simulink model "DCAC_conv_VSM"  (R2025a)
settings: Solver=VariableStepAuto  StartTime=0.0  StopTime=10.0  RelTol=1e-3
undefined symbols (not defined in the file): Cf, Fi, Grid_op_VCVSC, Grid_op_VSM, Grid_opDC_VSM, Grid_opVCVSC, Ki_w, Kic, Kiv, Kp_id, Kp_theta, Kp_w, Kpc, Kpv, Lc, Lf, mp, nq, Preffast, Rc, Rf, t_step, Tf, VI_L, VI_R, WOF_Tf
libraries: simulink x3
(part 3 of 3)

== system DCAC_conv_VSM/VSM/VCC/dynamic_limiting/VI/WOF_d ==
  In1 : Inport
  Gain : Gain  Gain=iTf
  I : Integrator  InitialConditionSource=external  InitialCondition=Grid_op_VCVSC.op.States(16).x'
  Sum : Sum  Inputs=+-|
  Sum4 : Sum  Inputs=|+-
  Out1 : Outport
  wires:
  Gain/1 -> I/1
  Sum4/1 -> Gain/1
  In1/1 -> I/2, Sum/1, Sum4/1
  I/1 -> Sum/2, Sum4/2
  Sum/1 -> Out1/1

== system DCAC_conv_VSM/VSM/VCC/dynamic_limiting/VI/WOF_q ==
  In1 : Inport
  Gain : Gain  Gain=iTf
  I : Integrator  InitialConditionSource=external  InitialCondition=Grid_op_VCVSC.op.States(17).x'
  Sum : Sum  Inputs=+-|
  Sum4 : Sum  Inputs=|+-
  Out1 : Outport
  wires:
  Gain/1 -> I/1
  Sum4/1 -> Gain/1
  In1/1 -> I/2, Sum/1, Sum4/1
  I/1 -> Sum/2, Sum4/2
  Sum/1 -> Out1/1

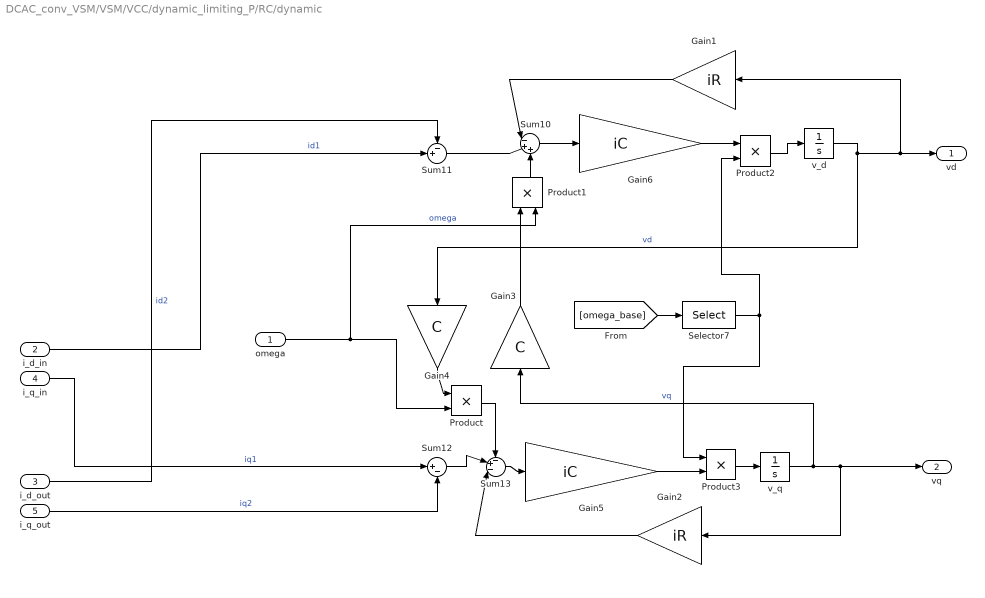
== system DCAC_conv_VSM/VSM/VCC/dynamic_limiting_P/RC/dynamic ==
  omega : Inport
  i_d_in : Inport  Port=2
  i_d_out : Inport  Port=3
  i_q_in : Inport  Port=4
  i_q_out : Inport  Port=5
  Gain1 : Gain  Gain=iR
  Gain2 : Gain  Gain=iR
  Gain3 : Gain  Gain=C
  Gain4 : Gain  Gain=C
  Gain5 : Gain  Gain=iC
  Gain6 : Gain  Gain=iC
  Product{,1..3} (4 alike) : Product
  Selector7 : Selector  InputPortWidth=length(fref.ref_units)  IndexOptions=Index vector (dialog)  Indices=block_fref  OutputSizes=1
  Sum10 : Sum  Inputs=|-++
  Sum11 : Sum  Inputs=-+|
  Sum12 : Sum  Inputs=|+-
  Sum13 : Sum  Inputs=-+-|
  v_d : Integrator  InitialCondition=Grid_opDC_VSM.vd_c
  v_q : Integrator  InitialCondition=Grid_opDC_VSM.vq_c
  vd : Outport
  vq : Outport  Port=2
  wires:
  Gain5/1 -> Product3/2
  Product3/1 -> v_q/1
  Selector7/1 -> Product3/1, Product2/2
  Product2/1 -> v_d/1
  Gain6/1 -> Product2/1
  [omega_base] -> Selector7/1
  i_q_out/1 -> Sum12/2  "iq2"
  i_q_in/1 -> Sum12/1  "iq1"
  i_d_out/1 -> Sum11/1  "id2"
  i_d_in/1 -> Sum11/2  "id1"
  v_d/1 -> Gain1/1, vd/1, Gain4/1  "vd"
  Sum12/1 -> Sum13/2
  Gain1/1 -> Sum10/1
  Sum13/1 -> Gain5/1
  omega/1 -> Product1/2, Product/2  "omega"
  Sum11/1 -> Sum10/2
  Product/1 -> Sum13/1
  Gain2/1 -> Sum13/3
  Gain4/1 -> Product/1
  Product1/1 -> Sum10/3
  v_q/1 -> Gain3/1, Gain2/1, vq/1  "vq"
  Gain3/1 -> Product1/1
  Sum10/1 -> Gain6/1

== system DCAC_conv_VSM/VSM/VCC/dynamic_limiting_P/RC/static ==
  omega : Inport
  i_d_in : Inport  Port=2
  i_d_out : Inport  Port=3
  i_q_in : Inport  Port=4
  i_q_out : Inport  Port=5
  Constant : Constant  Value=iR.^2
  Constant1 : Constant
  Divide : Product  Inputs=*/
  Gain : Gain  Gain=C
  Gain1 : Gain  Gain=iR
  Gain2 : Gain  Gain=iR
  Product{,1..5} (6 alike) : Product
  Sum : Sum  Inputs=|++
  Sum1 : Sum  Inputs=|-+
  Sum2 : Sum  Inputs=|+-
  Sum3 : Sum  Inputs=|++
  Sum4 : Sum  Inputs=|-+
  vd : Outport
  vq : Outport  Port=2
  wires:
  i_q_out/1 -> Sum2/2  "iq2"
  i_d_out/1 -> Sum2/1  "iq1"
  i_q_in/1 -> Sum1/1  "id2"
  i_d_in/1 -> Sum1/2  "id1"
  omega/1 -> Gain/1  "omega"
  Sum3/1 -> vd/1  "vd"
  Sum4/1 -> vq/1  "vq"
  Constant/1 -> Sum/1
  Sum/1 -> Divide/2
  Gain/1 -> Product2/2, Product/2, Product/1
  Product/1 -> Sum/2
  Constant1/1 -> Divide/1
  Sum1/1 -> Product1/1, Product4/1  "id"
  Sum2/1 -> Gain2/1, Product3/2  "iq"
  Gain1/1 -> Product1/2
  Divide/1 -> Product5/1, Gain1/1, Product2/1
  Product1/1 -> Sum3/1
  Product3/1 -> Sum3/2
  Product2/1 -> Product4/2, Product3/1
  Product4/1 -> Sum4/1
  Gain2/1 -> Product5/2
  Product5/1 -> Sum4/2

== system DCAC_conv_VSM/VSM/VCC/dynamic_limiting_P/RC/static omega ==
  i_d_in : Inport
  i_d_out : Inport  Port=2
  i_q_in : Inport  Port=3
  i_q_out : Inport  Port=4
  Gain : Gain  Gain=1./(iR.^2+C.^2)
  Gain2 : Gain  Gain=1./(iR.^2+C.^2)
  Gain3 : Gain  Gain=iR
  Gain4 : Gain  Gain=C
  Gain5 : Gain  Gain=iR
  Gain6 : Gain  Gain=C
  Sum : Sum  Inputs=|++
  Sum1 : Sum  Inputs=|+-
  Sum2 : Sum  Inputs=|+-
  Sum4 : Sum  Inputs=|-+
  vd : Outport
  vq : Outport  Port=2
  wires:
  Sum/1 -> vd/1
  Sum4/1 -> vq/1
  Gain5/1 -> Sum4/2
  Gain4/1 -> Sum4/1
  Gain6/1 -> Sum/2
  Gain3/1 -> Sum/1
  Gain2/1 -> Gain5/1, Gain6/1
  Gain/1 -> Gain3/1, Gain4/1
  i_d_out/1 -> Sum1/2
  i_d_in/1 -> Sum1/1  "id"
  i_q_out/1 -> Sum2/2  "iq2"
  Sum2/1 -> Gain2/1  "iq"
  Sum1/1 -> Gain/1  "id"
  i_q_in/1 -> Sum2/1  "iq1"

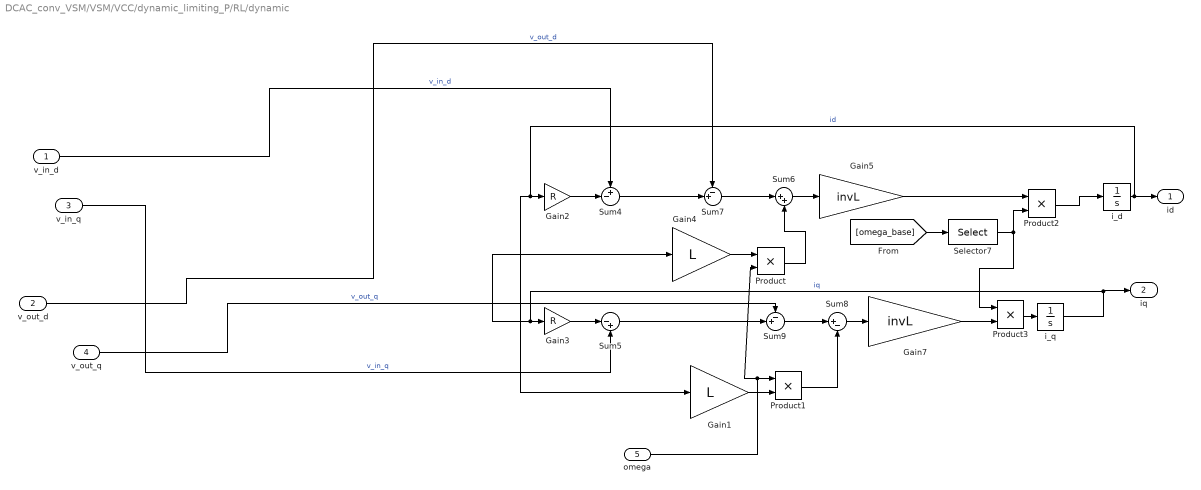
== system DCAC_conv_VSM/VSM/VCC/dynamic_limiting_P/RL/dynamic ==
  v_in_d : Inport
  v_out_d : Inport  Port=2
  v_in_q : Inport  Port=3
  v_out_q : Inport  Port=4
  omega : Inport  Port=5
  Gain1 : Gain  Gain=L
  Gain2 : Gain  Gain=R
  Gain3 : Gain  Gain=R
  Gain4 : Gain  Gain=L
  Gain5 : Gain  Gain=invL
  Gain7 : Gain  Gain=invL
  Product{,1..3} (4 alike) : Product
  Selector7 : Selector  InputPortWidth=length(fref.ref_units)  IndexOptions=Index vector (dialog)  Indices=block_fref  OutputSizes=1
  Sum4 : Sum  Inputs=+-|
  Sum5 : Sum  Inputs=|-+
  Sum6 : Sum  Inputs=|++
  Sum7 : Sum  Inputs=-+|
  Sum8 : Sum  Inputs=|+-
  Sum9 : Sum  Inputs=-+|
  i_d : Integrator  InitialCondition=Grid_opDC_VSM.id_l
  i_q : Integrator  InitialCondition=Grid_opDC_VSM.iq_l
  id : Outport
  iq : Outport  Port=2
  wires:
  Product3/1 -> i_q/1
  [omega_base] -> Selector7/1
  Selector7/1 -> Product3/1, Product2/2
  Product2/1 -> i_d/1
  Gain5/1 -> Product2/1
  omega/1 -> Product1/1, Product/2
  v_in_q/1 -> Sum5/2  "v_in_q"
  v_in_d/1 -> Sum4/1  "v_in_d"
  Gain2/1 -> Sum4/2
  i_d/1 -> Gain2/1, Gain1/1, id/1  "id"
  Sum6/1 -> Gain5/1
  Product/1 -> Sum6/2
  Sum8/1 -> Gain7/1
  Sum4/1 -> Sum7/2
  Product1/1 -> Sum8/2
  Gain4/1 -> Product/1
  Sum7/1 -> Sum6/1
  Gain3/1 -> Sum5/1
  Sum5/1 -> Sum9/2
  Gain7/1 -> Product3/2
  i_q/1 -> Gain3/1, Gain4/1, iq/1  "iq"
  Gain1/1 -> Product1/2
  Sum9/1 -> Sum8/1
  v_out_d/1 -> Sum7/1  "v_out_d"
  v_out_q/1 -> Sum9/1  "v_out_q"

== system DCAC_conv_VSM/VSM/VCC/dynamic_limiting_P/RL/static ==
  v_in_d : Inport
  v_out_d : Inport  Port=2
  v_in_q : Inport  Port=3
  v_out_q : Inport  Port=4
  omega : Inport  Port=5
  Constant : Constant  Value=R.^2
  Constant1 : Constant
  Divide : Product  Inputs=*/
  Gain : Gain  Gain=L
  Gain1 : Gain  Gain=R
  Gain2 : Gain  Gain=R
  Product{,1..5} (6 alike) : Product
  Sum : Sum  Inputs=|++
  Sum1 : Sum  Inputs=|+-
  Sum2 : Sum  Inputs=|+-
  Sum3 : Sum  Inputs=|++
  Sum4 : Sum  Inputs=|-+
  id : Outport
  iq : Outport  Port=2
  wires:
  v_in_q/1 -> Sum2/1  "v_in_q"
  v_out_d/1 -> Sum1/2  "v_out_d"
  Sum/1 -> Divide/2
  Gain2/1 -> Product5/2
  Product/1 -> Sum/2
  Product1/1 -> Sum3/1
  Product5/1 -> Sum4/2
  Constant/1 -> Sum/1
  Sum2/1 -> Product3/2, Product5/1  "vq"
  Gain/1 -> Product2/2, Product/1, Product/2
  Constant1/1 -> Divide/1
  Product3/1 -> Sum3/2
  Sum1/1 -> Product4/1, Product1/1  "vd"
  Divide/1 -> Product2/1, Gain1/1, Gain2/1
  Product4/1 -> Sum4/1
  Product2/1 -> Product3/1, Product4/2
  Gain1/1 -> Product1/2
  Sum3/1 -> id/1  "id"
  Sum4/1 -> iq/1  "iq"
  v_out_q/1 -> Sum2/2  "v_out_q"
  v_in_d/1 -> Sum1/1  "v_in_d"
  omega/1 -> Gain/1  "omega"

== system DCAC_conv_VSM/VSM/VCC/dynamic_limiting_P/RL/static_omega ==
  v_in_d : Inport
  v_out_d : Inport  Port=2
  v_in_q : Inport  Port=3
  v_out_q : Inport  Port=4
  Gain : Gain  Gain=1./(R.^2+L.^2)
  Gain2 : Gain  Gain=1./(R.^2+L.^2)
  Gain3 : Gain  Gain=R
  Gain4 : Gain  Gain=L
  Gain5 : Gain  Gain=L
  Gain6 : Gain  Gain=R
  Sum : Sum  Inputs=|++
  Sum1 : Sum  Inputs=|+-
  Sum2 : Sum  Inputs=|+-
  Sum3 : Sum  Inputs=|-+
  id : Outport
  iq : Outport  Port=2
  wires:
  Gain6/1 -> Sum3/2
  Sum3/1 -> iq/1
  Gain5/1 -> Sum3/1
  Sum/1 -> id/1
  Gain2/1 -> Gain4/1, Gain6/1
  Gain4/1 -> Sum/2
  Gain3/1 -> Sum/1
  Gain/1 -> Gain3/1, Gain5/1
  Sum2/1 -> Gain2/1  "vq"
  Sum1/1 -> Gain/1  "vd"
  v_out_d/1 -> Sum1/2  "v_out_d"
  v_out_q/1 -> Sum2/2  "v_out_q"
  v_in_d/1 -> Sum1/1  "v_in_d"
  v_in_q/1 -> Sum2/1  "v_in_q"

== system DCAC_conv_VSM/VSM/VCC/dynamic_limiting_P/VI/LPF_omega ==
  in : Inport
  Gain : Gain  Gain=10
  I : Integrator
  Sum4 : Sum  Inputs=|+-
  out : Outport
  wires:
  I/1 -> out/1, Sum4/2
  in/1 -> Sum4/1
  Sum4/1 -> Gain/1
  Gain/1 -> I/1

== system DCAC_conv_VSM/VSM/VCC/dynamic_limiting_P/VI/LPF_omega1 ==
  in : Inport
  Gain : Gain  Gain=10
  I : Integrator
  Sum4 : Sum  Inputs=|+-
  out : Outport
  wires:
  Gain/1 -> I/1
  Sum4/1 -> Gain/1
  in/1 -> Sum4/1
  I/1 -> Sum4/2, out/1

== system DCAC_conv_VSM/VSM/VCC/dynamic_limiting_P/VI/WOF_d ==
  In1 : Inport
  Gain : Gain  Gain=iTf
  I : Integrator  InitialConditionSource=external  InitialCondition=Grid_op_VCVSC.op.States(16).x'
  Sum : Sum  Inputs=+-|
  Sum4 : Sum  Inputs=|+-
  Out1 : Outport
  wires:
  Gain/1 -> I/1
  Sum4/1 -> Gain/1
  In1/1 -> I/2, Sum/1, Sum4/1
  I/1 -> Sum/2, Sum4/2
  Sum/1 -> Out1/1

== system DCAC_conv_VSM/VSM/VCC/dynamic_limiting_P/VI/WOF_q ==
  In1 : Inport
  Gain : Gain  Gain=iTf
  I : Integrator  InitialConditionSource=external  InitialCondition=Grid_op_VCVSC.op.States(17).x'
  Sum : Sum  Inputs=+-|
  Sum4 : Sum  Inputs=|+-
  Out1 : Outport
  wires:
  Gain/1 -> I/1
  Sum4/1 -> Gain/1
  In1/1 -> I/2, Sum/1, Sum4/1
  I/1 -> Sum/2, Sum4/2
  Sum/1 -> Out1/1
